simulink model "Third_order_Butterworth_filter"  (R2025a)
settings: Solver=VariableStepAuto  StartTime=0.0  StopTime=5  RelTol=1e-3
InitFcn:
  | Wn = 10;
  | T = 0.001;
undefined symbols (not defined in the file): dspblkCoreblockFVToolHelper, gcbh
settings Model: Creator=星必尘Sguan  LastModifiedBy=星必尘Sguan
settings SFSimCC: SimCustomHeaderCode="#include \"BPF_Loop.h\""  SimCustomInitializer=BPF_Init();  SimUserSources=BPF_Loop.c

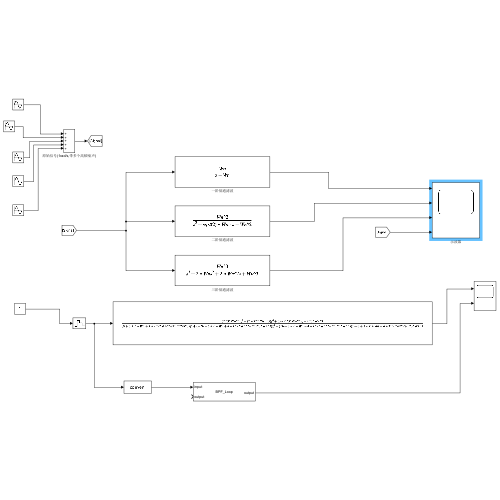
[thumbnail: Simulink's stored preview of the top-level diagram]
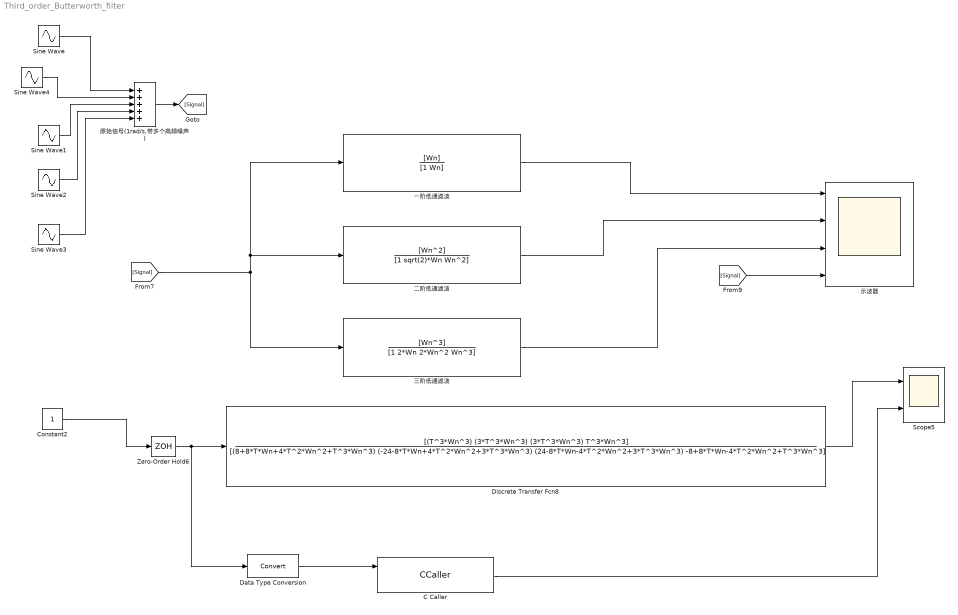
== system Third_order_Butterworth_filter ==
  C Caller : CCaller  FunctionName=BPF_Loop  PortSpecificationStruct="%)30     .    X ,   8    (     @         %    \"     (    !     0         %  0 \"0    $    _    07)G3F%M90  4&]R=$YA;64 4V-O<&4     26YD97@     5'EP90      4VEZ90      27-';&]B86P   X    X    !@    @    $          4    (     0    4    !         !     %    :6YP=70    .    .     8    (    !          %    \"     $    %     0         0    !0   &EN<'5T    #@   #@    &    \"     0         !0    @    !    !0    $         $     4   !);G!U=     X    X    !@    @    &          4    (     0    $    !          D    (               .    .     8    (    !          %    \"     $    &     0         0    !@   '-I;F=L90  #@   #     &    \"     0         !0    @    !     0    $         $  ! #$    .    ,     8    (    \"0(        %    \"     $    !     0         \"  $       X    X    !@    @    $          4    (     0    8    !         !     &    ;W5T<'5T   .    .     8    (    !          %    \"     $    &     0         0    !@   &]U='!U=   #@   $     &    \"     0         !0    @    !    \"P    $         $     L   !);G!U=$]U='!U=       #@   #@    &    \"     8         !0    @    !     0    $         \"0    @           #P/PX    X    !@    @    $          4    (     0    8    !         !     &    <VEN9VQE   .    ,     8    (    !          %    \"     $    \"     0         0  ( +3$   X    P    !@    @    ) @        4    (     0    $    !          (  0"
  Constant2 : Constant
  Data Type Conversion : DataTypeConversion  SaturateOnIntegerOverflow=off  RndMeth=Floor
  Discrete Transfer Fcn8 : DiscreteTransferFcn  LoadFcn=dspblkCoreblockFVToolHelper(gcbh,'load');  Numerator=[(T^3*Wn^3) (3*T^3*Wn^3) (3*T^3*Wn^3) T^3*Wn^3]  Denominator=[(8+8*T*Wn+4*T^2*Wn^2+T^3*Wn^3) (-24-8*T*Wn+4*T^2*Wn^2+3*T^3*Wn^3) (24-8*T*Wn-4*T^2*Wn^2+3*T^3*Wn^3) -8+8*T*Wn-4*T^2*Wn^2+T^3*Wn^3]
      settings: CopyFcn=dspblkCoreblockFVToolHelper(gcbh,'copy');  DeleteFcn=dspblkCoreblockFVToolHelper(gcbh,'close');  ModelCloseFcn=dspblkCoreblockFVToolHelper(gcbh,'close');  PreSaveFcn=dspblkCoreblockFVToolHelper(gcbh,'presave');  PostSaveFcn=dspblkCoreblockFVToolHelper(gcbh,'postsave');  CloseFcn=dspblkCoreblockFVToolHelper(gcbh,'close');
  Scope5 : Scope  NumInputPorts=2
      settings: ActiveDisplayYMinimum=-0.13403798128244301  ActiveDisplayYMaximum=1.2063430691042178  DataLoggingVariableName=ScopeData5
  Sine Wave : Sin  Amplitude=200  SampleTime=0
  Sine Wave1 : Sin  Amplitude=8  Frequency=50  SampleTime=0
  Sine Wave2 : Sin  Amplitude=6  Frequency=500  SampleTime=0
  Sine Wave3 : Sin  Amplitude=2  Frequency=2000  SampleTime=0
  Sine Wave4 : Sin  Amplitude=20  Frequency=24  SampleTime=0
  Zero-Order Hold6 : ZeroOrderHold  SampleTime=0.001
  一阶低通滤波 : TransferFcn  Numerator=[Wn]  Denominator=[1 Wn]
  三阶低通滤波 : TransferFcn  Numerator=[Wn^3]  Denominator=[1 2*Wn 2*Wn^2 Wn^3]
  二阶低通滤波 : TransferFcn  Numerator=[Wn^2]  Denominator=[1 sqrt(2)*Wn Wn^2]
  原始信号(1rad/s,带多个高频噪声) : Sum  Inputs=+++++
  示波器 : Scope  NumInputPorts=4
      settings: ActiveDisplayYMinimum=-289.523268507868  ActiveDisplayYMaximum=289.66750049431852  DataLoggingVariableName=ScopeData6
  wires:
  [Signal] -> 示波器/4
  [Signal] -> 三阶低通滤波/1, 二阶低通滤波/1, 一阶低通滤波/1
  一阶低通滤波/1 -> 示波器/1
  三阶低通滤波/1 -> 示波器/3
  二阶低通滤波/1 -> 示波器/2
  Constant2/1 -> Zero-Order Hold6/1
  C Caller/1 -> Scope5/2
  Discrete Transfer Fcn8/1 -> Scope5/1
  Zero-Order Hold6/1 -> Data Type Conversion/1, Discrete Transfer Fcn8/1
  Data Type Conversion/1 -> C Caller/1
  Sine Wave3/1 -> 原始信号(1rad/s,带多个高频噪声)/5
  Sine Wave4/1 -> 原始信号(1rad/s,带多个高频噪声)/2
  Sine Wave/1 -> 原始信号(1rad/s,带多个高频噪声)/1
  Sine Wave2/1 -> 原始信号(1rad/s,带多个高频噪声)/4
  原始信号(1rad/s,带多个高频噪声)/1 -> [Signal]
  Sine Wave1/1 -> 原始信号(1rad/s,带多个高频噪声)/3
